simulink model "parallelPID"  (R2024b)
settings: Solver=VariableStepAuto  StartTime=0.0  StopTime=10.0  RelTol=1e-3
values from neighbouring files (symbols this model uses):
  Kd = C.Kd    [helperscript.m]
  Ki = C.Ki    [helperscript.m]
  Kp = C.Kp    [helperscript.m]
  T_s = 0.01    [helperscript.m]
undefined symbols (not defined in the file or in its folder): classicModel, dspblkCoreblockFVToolHelper, gcbh
libraries: simulink x1
settings Model: Creator=dania  LastModifiedBy=domin

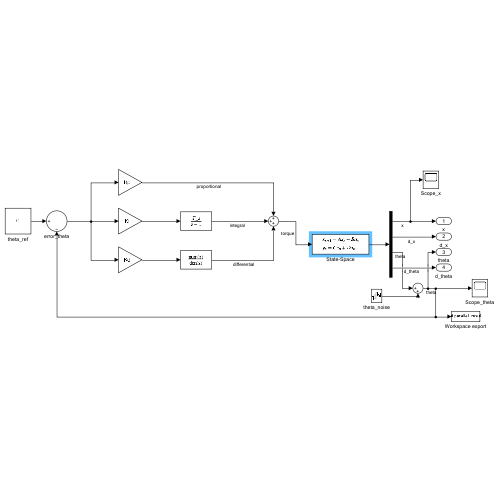
[thumbnail: Simulink's stored preview of the top-level diagram]
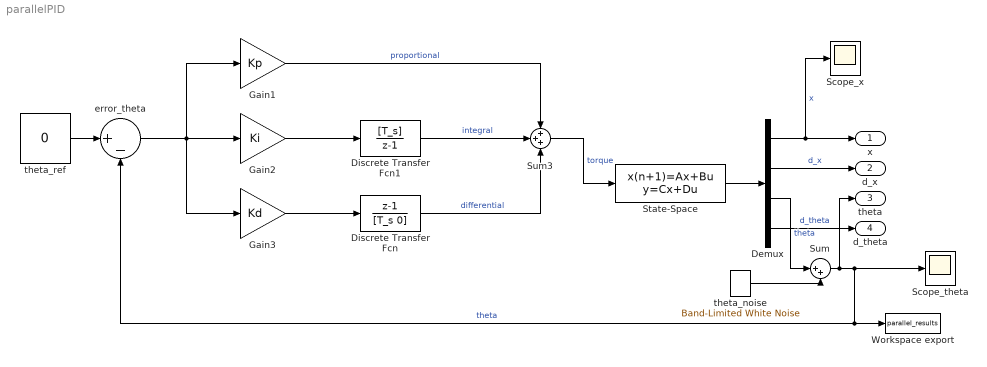
== system parallelPID ==
  Demux : Demux
  Discrete Transfer Fcn : DiscreteTransferFcn  LoadFcn=dspblkCoreblockFVToolHelper(gcbh,'load');  Numerator=[1 -1]  Denominator=[T_s 0]
      settings: CopyFcn=dspblkCoreblockFVToolHelper(gcbh,'copy');  DeleteFcn=dspblkCoreblockFVToolHelper(gcbh,'close');  ModelCloseFcn=dspblkCoreblockFVToolHelper(gcbh,'close');  PreSaveFcn=dspblkCoreblockFVToolHelper(gcbh,'presave');  PostSaveFcn=dspblkCoreblockFVToolHelper(gcbh,'postsave');  CloseFcn=dspblkCoreblockFVToolHelper(gcbh,'close');
  Discrete Transfer Fcn1 : DiscreteTransferFcn  LoadFcn=dspblkCoreblockFVToolHelper(gcbh,'load');  Numerator=[T_s]  Denominator=[1 -1]
      settings: CopyFcn=dspblkCoreblockFVToolHelper(gcbh,'copy');  DeleteFcn=dspblkCoreblockFVToolHelper(gcbh,'close');  ModelCloseFcn=dspblkCoreblockFVToolHelper(gcbh,'close');  PreSaveFcn=dspblkCoreblockFVToolHelper(gcbh,'presave');  PostSaveFcn=dspblkCoreblockFVToolHelper(gcbh,'postsave');  CloseFcn=dspblkCoreblockFVToolHelper(gcbh,'close');
  Gain1 : Gain  Gain=Kp
  Gain2 : Gain  Gain=Ki
  Gain3 : Gain  Gain=Kd
  Scope_theta : Scope
  Scope_x : Scope
  State-Space : DiscreteStateSpace  A=classicModel.A  B=classicModel.B  C=classicModel.C  D=classicModel.D  InitialCondition=[0;0;deg2rad(5);0]  SampleTime=0.01
  Sum : Sum  Inputs=|++
  Sum3 : Sum  Inputs=+++
  Workspace export : ToWorkspace  VariableName=parallel_results  SaveFormat=Structure With Time  SampleTime=-1
  error_theta : Sum  Inputs=|+-
  theta_noise : simulink/Sources/Band-Limited White Noise  Cov=[10^-9]  Ts=0.01  seed=[23341]
  theta_ref : Constant  Value=0
  x : Outport
  d_x : Outport  Port=2
  theta : Outport  Port=3
  d_theta : Outport  Port=4
  wires:
  theta_ref/1 -> error_theta/1
  error_theta/1 -> Gain1/1, Gain3/1, Gain2/1
  Discrete Transfer Fcn/1 -> Sum3/3  "differential"
  Demux/2 -> d_x/1  "d_x"
  State-Space/1 -> Demux/1
  Sum3/1 -> State-Space/1  "torque"
  Demux/1 -> Scope_x/1, x/1  "x"
  Gain1/1 -> Sum3/1  "proportional"
  Gain3/1 -> Discrete Transfer Fcn/1
  Gain2/1 -> Discrete Transfer Fcn1/1
  Discrete Transfer Fcn1/1 -> Sum3/2  "integral"
  Demux/4 -> d_theta/1  "d_theta"
  theta_noise/1 -> Sum/2
  Demux/3 -> Sum/1  "theta"
  Sum/1 -> theta/1, Scope_theta/1, Workspace export/1, error_theta/2  "theta"
